simulink model "ZCD"  (R2022b)
settings: Solver=FixedStepAuto  StartTime=0.0  StopTime=10.0  FixedStep=0.0001  RelTol=1e-3
settings Model: Creator=MAAM  LastModifiedBy=MAAM

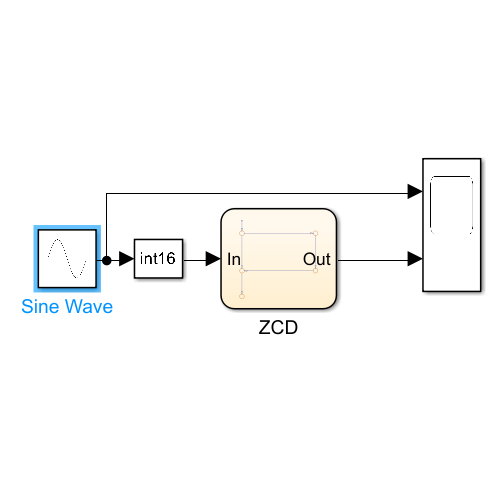
[thumbnail: Simulink's stored preview of the top-level diagram]
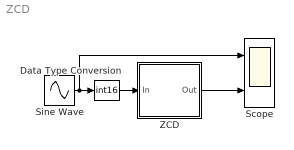
== system ZCD ==
  Data Type Conversion : DataTypeConversion  OutDataTypeStr=int16  SaturateOnIntegerOverflow=off  RndMeth=Floor
  Scope : Scope  NumInputPorts=2
  Sine Wave : Sin  Amplitude=220*sqrt(2)  Frequency=2 * pi * 5  SampleTime=0
  ZCD : Stateflow chart  TreatAsAtomicUnit=on
  wires:
  ZCD/1(Out) -> Scope/2
  Sine Wave/1 -> Scope/1, Data Type Conversion/1
  Data Type Conversion/1 -> ZCD/1(In)

== stateflow chart ZCD/ZCD ==
  (default) -> (junction 3)
  (junction 3) -> (junction 5) [order 1] : [hasChangedTo(In, 0)]
  (junction 3) -> (junction 9) [order 2] : {Out = 0;}
  (junction 5) -> (junction 7) : {Out = 1;}
  (junction 7) -> (junction 9)
  (junction 9) -> (junction 11)
  data: In input int16; Out output uint8
